simulink model "TEAM_6_MANUAL"  (R2020b)
settings: Solver=VariableStepAuto  StartTime=0.0  StopTime=10.0  RelTol=1e-3
libraries: simulink x2
settings Model: Creator=user  LastModifiedBy=99003740

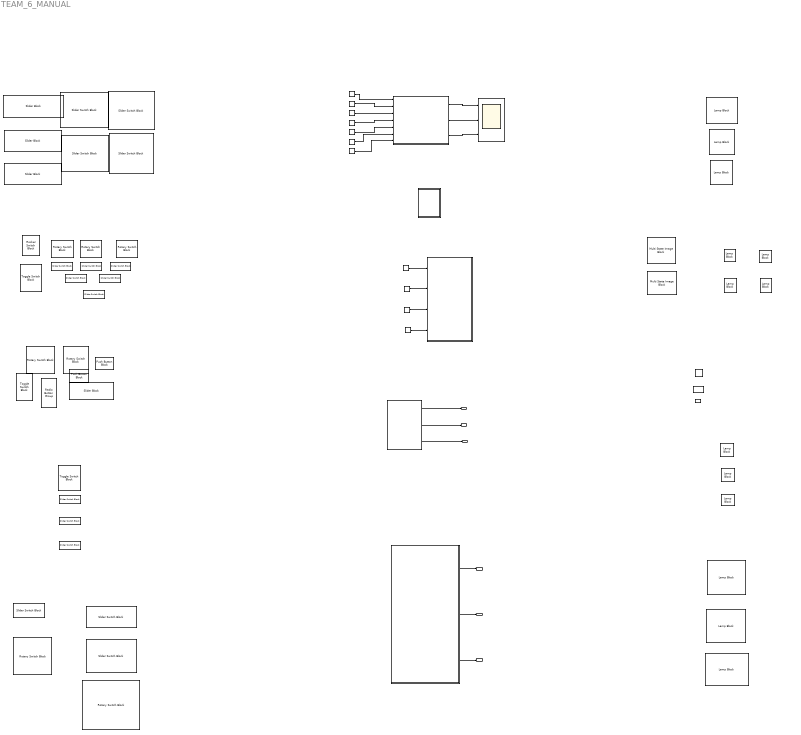
== system TEAM_6_MANUAL ==
  note: BCM_TEAM_6_HIL
  note: Wiper_band
  note: Dashboard
  note: KEY
  note: DASHBOARD
  note: DOME_LAMP
  note: Gray : Stop
      | Green : Very Slow
      | Blue : Normal Speed
      | Orange: Mid Speed
      | Yellow : High Speed
  note: BAT_Status
  note: Water_Spray
  note: Wiper
  note: Orange: Low BAT
      | Red : Very Low BAT
  note: READING_LAMP
  note: HVAC status Off
  note: WindShieldWiper
  note: Output Display
  note: Rear Fog removal OFF
  note: Air directed towards feet
  note: Air directed towards outlet
  note: Output Display
  note: HVAC status On
  note: Air directed towards windshield
  note: Recirculation
  note: Rear Fog removal ON
  " Passenger_Buckle" : SliderSwitchBlock
      settings: Values={{'Off', 'On'}, [0 1]}
  ACCESSORY : SliderSwitchBlock
      settings: Values={{'Off', 'On'}, [0 1]}
  BRIGHTNESS_BUTTON : RotarySwitchBlock
      settings: Values={{'Off', 'Low', 'Medium', 'High', 'very high'}, [0 1 2 3 4]}
  Bat : Constant  Value=24
  Controller : Subsystem
  DASHBOARD : LampBlock
  DOMELAMP : LampBlock
  DOME_BUTTON : SliderSwitchBlock
      settings: Values={{'Off', 'On'}, [0 1]}
  DOOR : RotarySwitchBlock
      settings: Values={{'Close', 'Door', 'Open'}, [0 1 2]}
  Driver remainder : LampBlock
  Driver_Buckle : SliderSwitchBlock
      settings: Values={{'Off', 'On'}, [0 1]}
  Front crash : Constant  Value=89.87630208333334
  Gear : Constant
  KEY : Constant  Value=0
  Lamp{,1..6} (7 alike) : LampBlock
  Lamp7 : LampBlock  LabelPosition=Hide
  Lamp8 : LampBlock  LabelPosition=Hide
  Lamp9 : LampBlock  LabelPosition=Hide
  MultiStateImage : MultiStateImageBlock
  MultiStateImage1 : MultiStateImageBlock
  Passenger Remainder : LampBlock
  Push Button : PushButtonBlock  LabelPosition=Bottom  ButtonText=Spray
  Push Button1 : PushButtonBlock  ButtonText=1X_Wiper
  READING_LAMP : LampBlock
  READLIGHT_BUTTON : SliderSwitchBlock
      settings: Values={{'Off', 'On'}, [0 1]}
  Radio Button : RadioButtonGroup  LabelPosition=Hide  SelectedLabel=P  ButtonGroupName=Gear_Box
      settings: Values={{'P', 'R', 'N', 'D', 'L'}, [1 2 0 3 4]}
  Rocker Switch : RockerSwitchBlock
      settings: Values={{'On', 'Off'}, [1 0]}
  Roll   Over : Constant  Value=73.98290094339622
  Rotary Switch : RotarySwitchBlock
      settings: Values={{'Off', 'Low', 'Medium', 'High'}, [0 1 2 3]}
  Rotary Switch1 : RotarySwitchBlock
      settings: Values={{'Off', 'Low', 'Medium', 'High'}, [0 1 2 3]}
  Rotary Switch2 : RotarySwitchBlock
      settings: Values={{'Off', 'AC', 'Heater', 'Air-Vent'}, [0 1 2 3]}
  Rotary Switch3 : RotarySwitchBlock  LabelPosition=Hide
      settings: Values={{'OFF', '-', 'NR', 'LO', 'HI'}, [0 1 2 3 4]}
  Rotary Switch4 : RotarySwitchBlock  LabelPosition=Hide
      settings: Values={{'OFF', 'ACC', 'IGNI'}, [0 1 2]}
  Scope1 : Scope  NumInputPorts=3
  Seatbelt{1..4} (4 alike) : Constant
  Side crash : Constant  Value=67.95726102941177
  Slider : SliderBlock
  Slider Switch{,1..6,9..12} (11 alike) : SliderSwitchBlock
      settings: Values={{'Off', 'On'}, [0 1]}
  Slider1 : SliderBlock
  Slider2 : SliderBlock
  Slider3 : SliderBlock  LabelPosition=Hide  ScaleMin=12  ScaleMax=24  TickInterval=6
  Subsystem1 : Subsystem
  Subsystem3 : Subsystem
  Subsystem4 : Subsystem
  Subsystem5 : Subsystem
  T_switch : Constant  Value=0
  Toggle Switch : ToggleSwitchBlock
      settings: Values={{'Off', 'On'}, [0 1]}
  Toggle Switch1 : ToggleSwitchBlock  LabelPosition=Hide
      settings: Values={{'TG_Close', 'TG_Open'}, [0 1]}
  Toggle Switch2 : ToggleSwitchBlock
      settings: Values={{'Off', 'On'}, [0 1]}
  Vehicle State : LampBlock
  Outport : Outport
  Outport1 : Outport  Port=2
  Outport2 : Outport  Port=3
  DL : Outport  Port=4
  dash_light : Outport  Port=5
  reading_lamp : Outport  Port=6
  wires:
  Side crash/1 -> Subsystem1/2(In2)
  Front crash/1 -> Subsystem1/1(In1)
  Seatbelt2/1 -> Subsystem1/5(Inport4)
  Subsystem1/3(All Airbag) -> Scope1/3
  Roll   Over/1 -> Subsystem1/3(Inport2)
  Seatbelt3/1 -> Subsystem1/6(Inport5)
  Seatbelt4/1 -> Subsystem1/7(Inport6)
  Subsystem1/2(Airbag Side) -> Scope1/2
  Seatbelt1/1 -> Subsystem1/4(Inport3)
  Subsystem1/1(Airbag front) -> Scope1/1
  Gear/1 -> Controller/2(GEAR)
  Bat/1 -> Controller/3(BAT)
  T_switch/1 -> Controller/4(T_Switch)
  KEY/1 -> Controller/1(KEY)
  Subsystem4/1(Outport) -> Outport/1
  Subsystem4/2(Outport1) -> Outport1/1
  Subsystem4/3(Outport2) -> Outport2/1
  Subsystem5/1(DL) -> DL/1
  Subsystem5/3(reading_lamp) -> reading_lamp/1
  Subsystem5/2(dash_light) -> dash_light/1

== system TEAM_6_MANUAL/Controller ==
  note: Wiper_system
  note: TailGate_System
  KEY : Inport
  GEAR : Inport  Port=2
  BAT : Inport  Port=3
  T_Switch : Inport  Port=4
  Tail_Gate : Subsystem
  Wiper_System : Subsystem
  wires:
  KEY/1 -> Wiper_System/2(KEY), Tail_Gate/1(KEY)
  GEAR/1 -> Tail_Gate/3(GEAR)  "gear"
  BAT/1 -> Tail_Gate/2(BAT), Wiper_System/1(BAT)  "bat"
  T_Switch/1 -> Tail_Gate/4(T_Switch)  "t_swiitch"

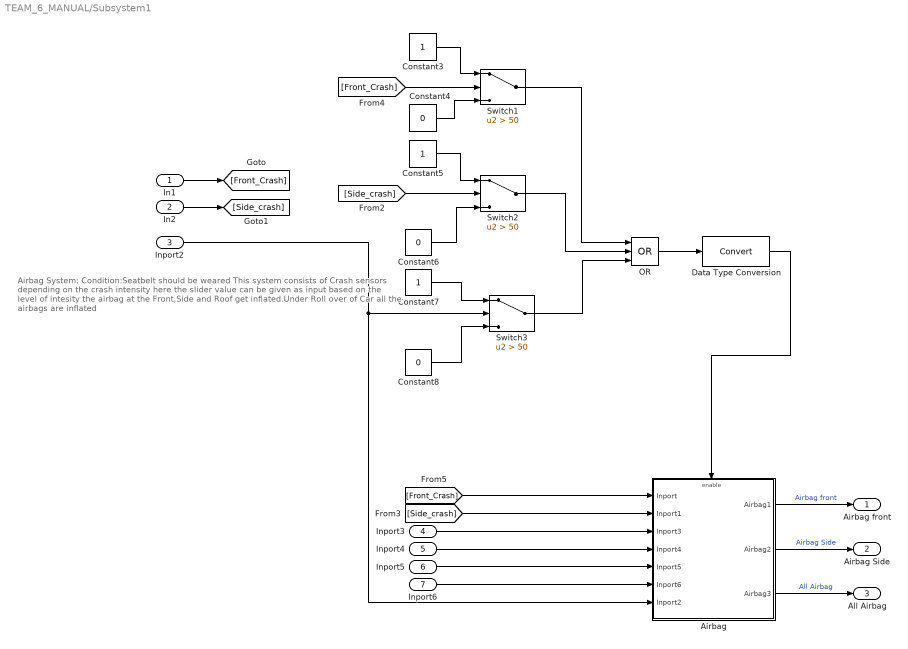
== system TEAM_6_MANUAL/Subsystem1 ==
  note: Airbag System:
      | Condition:Seatbelt should be weared
      | This system consists of Crash sensors depending on the
      | crash intensity here the slider value can be given as input
      | based on the level of intesity the airbag at the Front,Side and Roof get
      | inflated.Under Roll over of Car all the airbags are inflated
  In1 : Inport
  In2 : Inport  Port=2
  Inport2 : Inport  Port=3
  Inport3 : Inport  Port=4
  Inport4 : Inport  Port=5
  Inport5 : Inport  Port=6
  Inport6 : Inport  Port=7
  Airbag : Subsystem  TreatAsAtomicUnit=on
  Constant3 : Constant
  Constant4 : Constant  Value=0
  Constant5 : Constant
  Constant6 : Constant  Value=0
  Constant7 : Constant
  Constant8 : Constant  Value=0
  Data Type Conversion : DataTypeConversion
  OR : Logic  Operator=OR  Inputs=3  IconShape=distinctive  AllPortsSameDT=off  OutDataTypeStr=boolean
  Switch1 : Switch  Criteria=u2 > Threshold  Threshold=50
  Switch2 : Switch  Criteria=u2 > Threshold  Threshold=50
  Switch3 : Switch  Criteria=u2 > Threshold  Threshold=50
  Airbag front : Outport
  Airbag Side : Outport  Port=2
  All Airbag : Outport  Port=3
  wires:
  Constant7/1 -> Switch3/1
  Constant6/1 -> Switch2/3
  Switch3/1 -> OR/3
  Switch2/1 -> OR/2
  Airbag/3(Airbag3) -> All Airbag/1  "All Airbag"
  Airbag/2(Airbag2) -> Airbag Side/1  "Airbag Side"
  Inport6/1 -> Airbag/6(Inport6)
  OR/1 -> Data Type Conversion/1
  Inport4/1 -> Airbag/4(Inport4)
  Inport5/1 -> Airbag/5(Inport5)
  Inport2/1 -> Airbag/7(Inport2), Switch3/2
  In2/1 -> [Side_crash]
  [Side_crash] -> Airbag/2(Inport1)
  Constant4/1 -> Switch1/3
  [Front_Crash] -> Switch1/2
  [Front_Crash] -> Airbag/1(Inport)
  [Side_crash] -> Switch2/2
  Data Type Conversion/1 -> Airbag/Enable
  Constant3/1 -> Switch1/1
  In1/1 -> [Front_Crash]
  Switch1/1 -> OR/1
  Constant8/1 -> Switch3/3
  Constant5/1 -> Switch2/1
  Inport3/1 -> Airbag/3(Inport3)
  Airbag/1(Airbag1) -> Airbag front/1  "Airbag front"

== system TEAM_6_MANUAL/Subsystem3 ==
  note: HVAC SYSTEM
      |
      | Des cription:
  Hood and HVAC Subsystem : Subsystem  TreatAsAtomicUnit=on

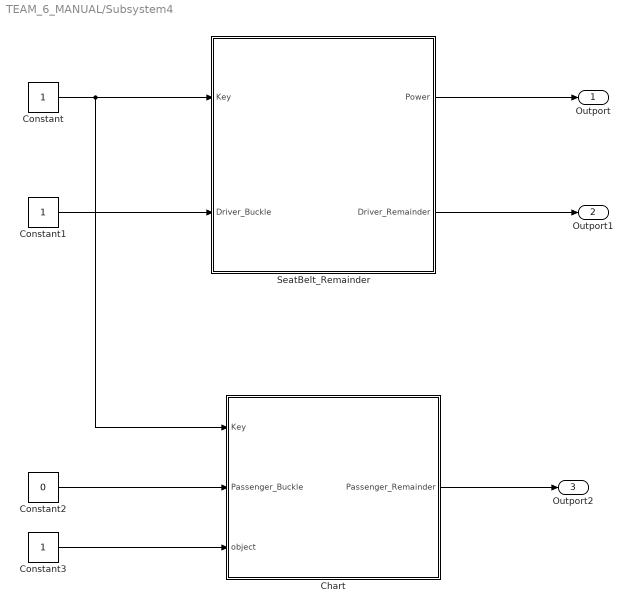
== system TEAM_6_MANUAL/Subsystem4 ==
  Chart : Stateflow chart  TreatAsAtomicUnit=on
  Constant : Constant
  Constant1 : Constant
  Constant2 : Constant  Value=0
  Constant3 : Constant
  SeatBelt_Remainder : Stateflow chart  TreatAsAtomicUnit=on
  Outport : Outport
  Outport1 : Outport  Port=2
  Outport2 : Outport  Port=3
  wires:
  Constant/1 -> Chart/1(Key), SeatBelt_Remainder/1(Key)
  SeatBelt_Remainder/1(Power) -> Outport/1
  SeatBelt_Remainder/2(Driver_Remainder) -> Outport1/1
  Constant1/1 -> SeatBelt_Remainder/2(Driver_Buckle)
  Constant2/1 -> Chart/2(Passenger_Buckle)
  Constant3/1 -> Chart/3(object)
  Chart/1(Passenger_Remainder) -> Outport2/1

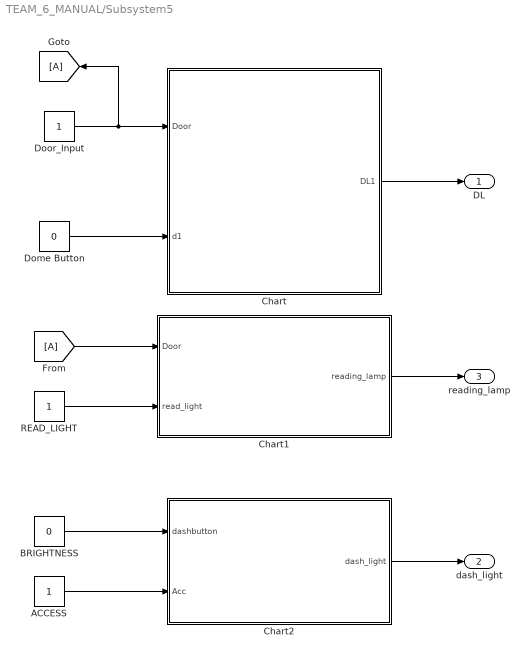
== system TEAM_6_MANUAL/Subsystem5 ==
  ACCESS : Constant
  BRIGHTNESS : Constant  Value=0
  Chart : Stateflow chart  TreatAsAtomicUnit=on
  Chart1 : Stateflow chart  TreatAsAtomicUnit=on
  Chart2 : Stateflow chart  TreatAsAtomicUnit=on
  Dome Button : Constant  Value=0
  Door_Input : Constant
  READ_LIGHT : Constant
  DL : Outport
  dash_light : Outport  Port=2
  reading_lamp : Outport  Port=3
  wires:
  Chart1/1(reading_lamp) -> reading_lamp/1
  Door_Input/1 -> Chart/1(Door), [A]
  [A] -> Chart1/1(Door)
  BRIGHTNESS/1 -> Chart2/1(dashbutton)
  ACCESS/1 -> Chart2/2(Acc)
  Chart2/1(dash_light) -> dash_light/1
  Chart/1(DL1) -> DL/1
  Dome Button/1 -> Chart/2(d1)
  READ_LIGHT/1 -> Chart1/2(read_light)

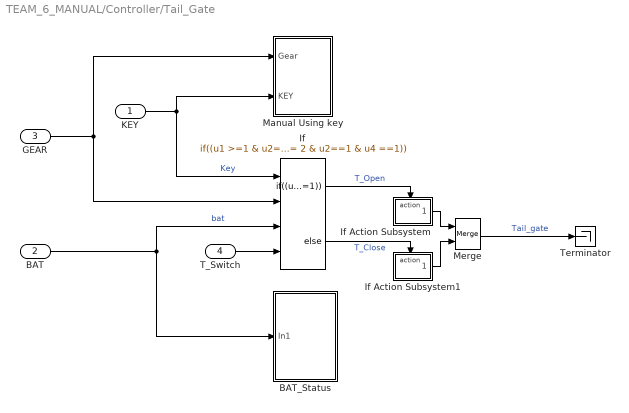
== system TEAM_6_MANUAL/Controller/Tail_Gate ==
  KEY : Inport
  BAT : Inport  Port=2
  GEAR : Inport  Port=3
  T_Switch : Inport  Port=4
  BAT_Status : Subsystem
  If : If  NumInputs=4  IfExpression=(u1 >=1 & u2==1 & u3 >20 & u4 ==1)|(u1 == 2 & u2==1 & u4 ==1)
  If Action Subsystem : Subsystem  TreatAsAtomicUnit=on
  If Action Subsystem1 : Subsystem  TreatAsAtomicUnit=on
  Manual Using key : Subsystem
  Merge : Merge
  Terminator : Terminator
  wires:
  If/1 -> If Action Subsystem/Action  "T_Open"
  BAT/1 -> If/3, BAT_Status/1(In1)  "bat"
  KEY/1 -> Manual Using key/2(KEY), If/1  "Key"
  GEAR/1 -> Manual Using key/1(Gear), If/2
  If Action Subsystem/1(Inport) -> Merge/1
  If/2 -> If Action Subsystem1/Action  "T_Close"
  If Action Subsystem1/1(Inport) -> Merge/2
  Merge/1 -> Terminator/1  "Tail_gate"
  T_Switch/1 -> If/4

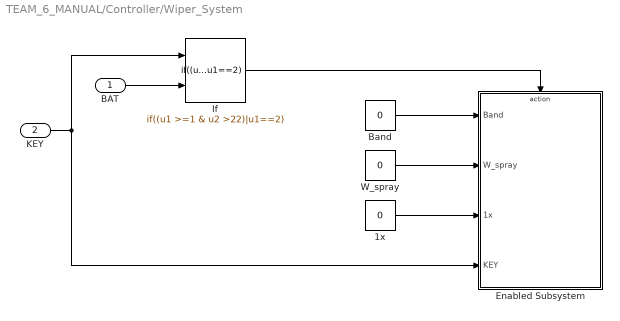
== system TEAM_6_MANUAL/Controller/Wiper_System ==
  BAT : Inport
  KEY : Inport  Port=2
  1x : Constant  Value=0
  Band : Constant  Value=0
  Enabled Subsystem : Subsystem  TreatAsAtomicUnit=on
  If : If  NumInputs=2  IfExpression=(u1 >=1 & u2 >22)|u1==2  ShowElse=off
  W_spray : Constant  Value=0
  wires:
  If/1 -> Enabled Subsystem/Action
  W_spray/1 -> Enabled Subsystem/2(W_spray)
  Band/1 -> Enabled Subsystem/1(Band)
  KEY/1 -> If/1, Enabled Subsystem/4(KEY)
  1x/1 -> Enabled Subsystem/3(1x)
  BAT/1 -> If/2

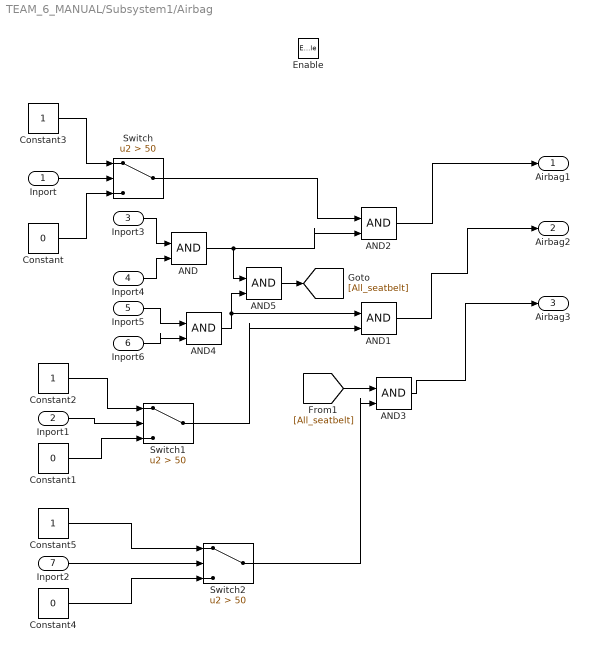
== system TEAM_6_MANUAL/Subsystem1/Airbag ==
  Inport : Inport
  Inport1 : Inport  Port=2
  Inport3 : Inport  Port=3
  Inport4 : Inport  Port=4
  Inport5 : Inport  Port=5
  Inport6 : Inport  Port=6
  Inport2 : Inport  Port=7
  Enable : EnablePort
  AND{,1..5} (6 alike) : Logic  IconShape=distinctive  AllPortsSameDT=off  OutDataTypeStr=boolean
  Constant : Constant  Value=0
  Constant1 : Constant  Value=0
  Constant2 : Constant
  Constant3 : Constant
  Constant4 : Constant  Value=0
  Constant5 : Constant
  Switch : Switch  Criteria=u2 > Threshold  Threshold=50
  Switch1 : Switch  Criteria=u2 > Threshold  Threshold=50
  Switch2 : Switch  Criteria=u2 > Threshold  Threshold=50
  Airbag1 : Outport
  Airbag2 : Outport  Port=2
  Airbag3 : Outport  Port=3
  wires:
  Constant2/1 -> Switch1/1
  Inport/1 -> Switch/2
  Constant/1 -> Switch/3
  Inport1/1 -> Switch1/2
  Constant1/1 -> Switch1/3
  Constant3/1 -> Switch/1
  Switch/1 -> AND2/1
  AND2/1 -> Airbag1/1
  AND1/1 -> Airbag2/1
  AND3/1 -> Airbag3/1
  Inport3/1 -> AND/1
  Inport4/1 -> AND/2
  Inport5/1 -> AND4/1
  Inport6/1 -> AND4/2
  Constant4/1 -> Switch2/3
  Inport2/1 -> Switch2/2
  Constant5/1 -> Switch2/1
  AND/1 -> AND5/1, AND2/2
  AND4/1 -> AND1/1, AND5/2
  Switch1/1 -> AND1/2
  AND5/1 -> [All_seatbelt]
  [All_seatbelt] -> AND3/1
  Switch2/1 -> AND3/2

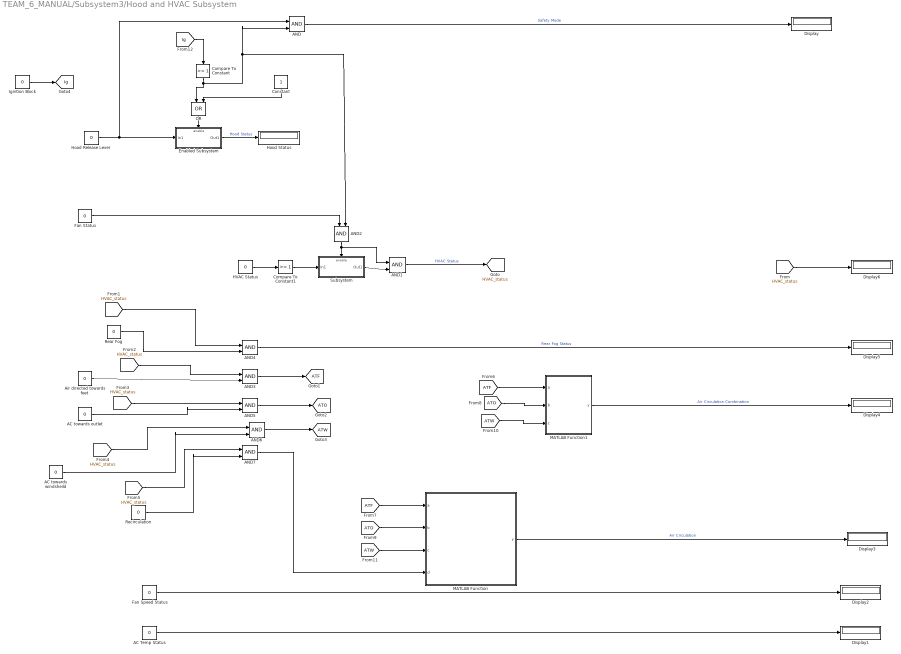
== system TEAM_6_MANUAL/Subsystem3/Hood and HVAC Subsystem ==
  AC Temp Status : Constant  Value=0
  AC towards outlet : Constant  Value=0
  AC towards windsheild : Constant  Value=0
  AND{,1..7} (8 alike) : Logic  IconShape=distinctive  AllPortsSameDT=off  OutDataTypeStr=boolean
  Air directed towards feet : Constant  Value=0
  Compare To Constant : simulink/Logic and Bit Operations/Compare To Constant  relop=>=  const=1  OutDataTypeStr=boolean
  Compare To Constant1 : simulink/Logic and Bit Operations/Compare To Constant  relop=>=  const=1  OutDataTypeStr=boolean
  Constant : Constant
  Display{,1..6} (7 alike) : Display
  Enabled Subsystem : Subsystem  TreatAsAtomicUnit=on
  Fan Speed Status : Constant  Value=0
  Fan Status : Constant  Value=0
  HVAC Status : Constant  Value=0
  Hood Release Lever : Constant  Value=0
  Hood Status : Display
  Ignition Block : Constant  Value=0
  MATLAB Function : MATLAB Function  TreatAsAtomicUnit=on
  MATLAB Function1 : MATLAB Function  TreatAsAtomicUnit=on
  OR : Logic  Operator=OR  IconShape=distinctive  AllPortsSameDT=off  OutDataTypeStr=boolean
  Rear Fog : Constant  Value=0
  Recirculation : Constant  Value=0
  Subsystem : Subsystem
  tag scope: ATF=global, ATO=global, ATW=global, HVAC_status=global, Ig=global
  wires:
  AND/1 -> Display/1  "Safety Mode"
  Hood Release Lever/1 -> Enabled Subsystem/1(In1), AND/1
  Compare To Constant/1 -> AND2/2, AND/2, OR/1
  OR/1 -> Enabled Subsystem/Enable
  Enabled Subsystem/1(Out1) -> Hood Status/1  "Hood Status"
  Constant/1 -> OR/2
  AND1/1 -> [HVAC_status]  "HVAC Status"
  Subsystem/1(Out1) -> AND1/2
  AND2/1 -> AND1/1, Subsystem/Enable
  Compare To Constant1/1 -> Subsystem/1(In1)
  HVAC Status/1 -> Compare To Constant1/1
  Recirculation/1 -> AND7/2
  AND4/1 -> Display5/1  "Rear Fog Status"
  Rear Fog/1 -> AND4/2
  AC towards outlet/1 -> AND5/2
  Air directed towards feet/1 -> AND3/2
  AC towards windsheild/1 -> AND6/2
  MATLAB Function/1(y) -> Display3/1  "Air Circulation"
  AND7/1 -> MATLAB Function/4(d)
  MATLAB Function1/1(y) -> Display4/1  "Air Circulation Combination"
  AC Temp Status/1 -> Display1/1
  Fan Speed Status/1 -> Display2/1
  Fan Status/1 -> AND2/1
  [HVAC_status] -> Display6/1
  [HVAC_status] -> AND4/1
  [HVAC_status] -> AND3/1
  [HVAC_status] -> AND5/1
  [HVAC_status] -> AND6/1
  [HVAC_status] -> AND7/1
  AND3/1 -> [ATF]
  [ATF] -> MATLAB Function1/1(a)
  [ATF] -> MATLAB Function/1(a)
  AND5/1 -> [ATO]
  [ATO] -> MATLAB Function1/2(b)
  [ATO] -> MATLAB Function/2(b)
  AND6/1 -> [ATW]
  [ATW] -> MATLAB Function1/3(c)
  [ATW] -> MATLAB Function/3(c)
  Ignition Block/1 -> [Ig]
  [Ig] -> Compare To Constant/1

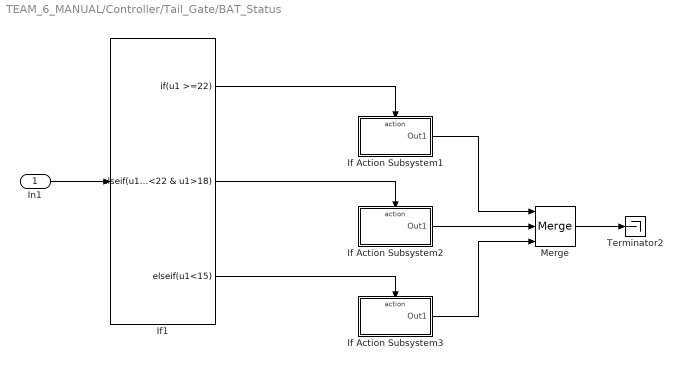
== system TEAM_6_MANUAL/Controller/Tail_Gate/BAT_Status ==
  In1 : Inport
  If Action Subsystem1 : Subsystem  TreatAsAtomicUnit=on
  If Action Subsystem2 : Subsystem  TreatAsAtomicUnit=on
  If Action Subsystem3 : Subsystem  TreatAsAtomicUnit=on
  If1 : If  IfExpression=u1 >=22  ElseIfExpressions=u1<22 & u1>18, u1<15  ShowElse=off
  Merge : Merge  Inputs=3
  Terminator2 : Terminator
  wires:
  In1/1 -> If1/1
  If Action Subsystem1/1(Out1) -> Merge/1
  Merge/1 -> Terminator2/1
  If1/1 -> If Action Subsystem1/Action
  If1/2 -> If Action Subsystem2/Action
  If Action Subsystem3/1(Out1) -> Merge/3
  If1/3 -> If Action Subsystem3/Action
  If Action Subsystem2/1(Out1) -> Merge/2

== system TEAM_6_MANUAL/Controller/Tail_Gate/If Action Subsystem ==
  Action Port : ActionPort  ActionPortLabel=if((u1 >=1 & u2==1 & u3 >20 & u4 ==1)|(u1 == 2 & u2==1 & u4 ==1))
  Constant : Constant
  Inport : Outport
  wires:
  Constant/1 -> Inport/1

== system TEAM_6_MANUAL/Controller/Tail_Gate/If Action Subsystem1 ==
  Action Port : ActionPort  ActionPortLabel=else
  Constant : Constant  Value=0
  Inport : Outport
  wires:
  Constant/1 -> Inport/1

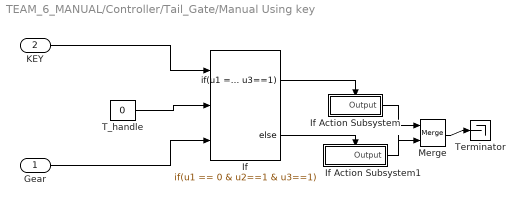
== system TEAM_6_MANUAL/Controller/Tail_Gate/Manual Using key ==
  Gear : Inport
  KEY : Inport  Port=2
  If : If  NumInputs=3  IfExpression=u1 == 0 & u2==1 & u3==1
  If Action Subsystem : Subsystem  TreatAsAtomicUnit=on
  If Action Subsystem1 : Subsystem  TreatAsAtomicUnit=on
  Merge : Merge
  T_handle : Constant  Value=0
  Terminator : Terminator
  wires:
  KEY/1 -> If/1
  If Action Subsystem/1(Output) -> Merge/1
  If/1 -> If Action Subsystem/Action
  If Action Subsystem1/1(Output) -> Merge/2
  If/2 -> If Action Subsystem1/Action
  Merge/1 -> Terminator/1
  T_handle/1 -> If/2
  Gear/1 -> If/3

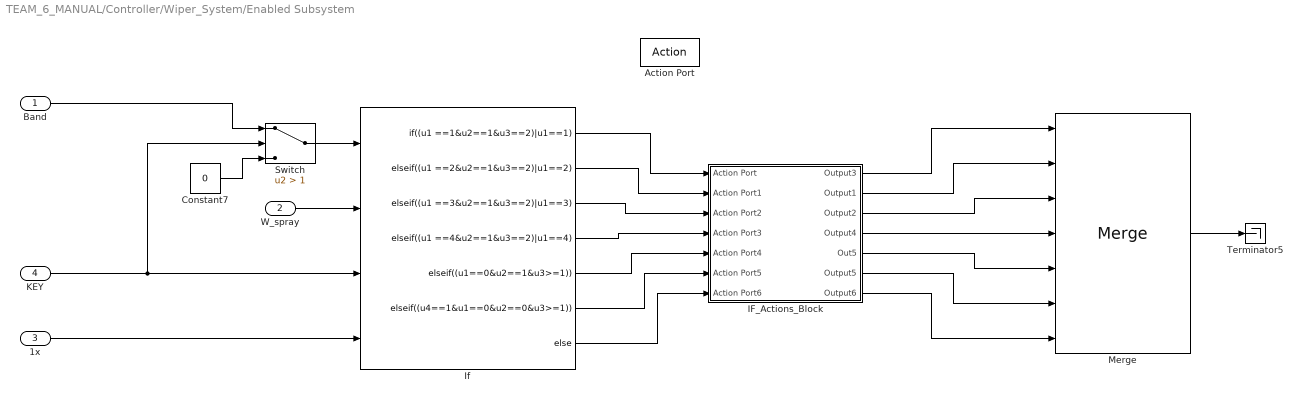
== system TEAM_6_MANUAL/Controller/Wiper_System/Enabled Subsystem ==
  Band : Inport
  W_spray : Inport  Port=2
  1x : Inport  Port=3
  KEY : Inport  Port=4
  Action Port : ActionPort  ActionPortLabel=if((u1 >=1 & u2 >22)|u1==2)
  Constant7 : Constant  Value=0
  IF_Actions_Block : Subsystem
  If : If  NumInputs=4  IfExpression=(u1 ==1&u2==1&u3==2)|u1==1  ElseIfExpressions=(u1 ==2&u2==1&u3==2)|u1==2,(u1 ==3&u2==1&u3==2)|u1==3,(u1 ==4&u2==1&u3==2)|u1==4,(u1==0&u2==1&u3>=1),(u4==1&u1==0&u2==0&u3>=1)
  Merge : Merge  Inputs=7
  Switch : Switch  Criteria=u2 > Threshold  Threshold=1
  Terminator5 : Terminator
  wires:
  Merge/1 -> Terminator5/1
  W_spray/1 -> If/2
  1x/1 -> If/4
  KEY/1 -> Switch/2, If/3
  Switch/1 -> If/1
  Band/1 -> Switch/1
  Constant7/1 -> Switch/3
  If/1 -> IF_Actions_Block/1(Action Port)
  If/2 -> IF_Actions_Block/2(Action Port1)
  If/3 -> IF_Actions_Block/3(Action Port2)
  If/4 -> IF_Actions_Block/4(Action Port3)
  If/5 -> IF_Actions_Block/5(Action Port4)
  If/6 -> IF_Actions_Block/6(Action Port5)
  If/7 -> IF_Actions_Block/7(Action Port6)
  IF_Actions_Block/1(Output3) -> Merge/1
  IF_Actions_Block/2(Output1) -> Merge/2
  IF_Actions_Block/3(Output2) -> Merge/3
  IF_Actions_Block/4(Output4) -> Merge/4
  IF_Actions_Block/5(Out5) -> Merge/5
  IF_Actions_Block/6(Output5) -> Merge/6
  IF_Actions_Block/7(Output6) -> Merge/7

== system TEAM_6_MANUAL/Subsystem3/Hood and HVAC Subsystem/Enabled Subsystem ==
  In1 : Inport
  Enable : EnablePort
  Out1 : Outport  InitialOutput=0  VectorParamsAs1DForOutWhenUnconnected=off
  wires:
  In1/1 -> Out1/1

== system TEAM_6_MANUAL/Subsystem3/Hood and HVAC Subsystem/Subsystem ==
  In1 : Inport
  Enable : EnablePort
  Out1 : Outport
  wires:
  In1/1 -> Out1/1

== system TEAM_6_MANUAL/Controller/Tail_Gate/BAT_Status/If Action Subsystem1 ==
  Action Port : ActionPort  ActionPortLabel=if(u1 >=22)
  Constant : Constant
  Out1 : Outport
  wires:
  Constant/1 -> Out1/1

== system TEAM_6_MANUAL/Controller/Tail_Gate/BAT_Status/If Action Subsystem2 ==
  Action Port : ActionPort  ActionPortLabel=elseif(u1<22 & u1>18)
  Constant : Constant  Value=2
  Out1 : Outport
  wires:
  Constant/1 -> Out1/1

== system TEAM_6_MANUAL/Controller/Tail_Gate/BAT_Status/If Action Subsystem3 ==
  Action Port : ActionPort  ActionPortLabel=elseif( u1<15)
  Constant : Constant  Value=3
  Out1 : Outport
  wires:
  Constant/1 -> Out1/1

== system TEAM_6_MANUAL/Controller/Tail_Gate/Manual Using key/If Action Subsystem ==
  Action Port : ActionPort  ActionPortLabel=if(u1 == 0 & u2==1 & u3==1)
  Constant2 : Constant
  Output : Outport
  wires:
  Constant2/1 -> Output/1

== system TEAM_6_MANUAL/Controller/Tail_Gate/Manual Using key/If Action Subsystem1 ==
  Action Port : ActionPort  ActionPortLabel=else
  Constant3 : Constant  Value=0
  Output : Outport
  wires:
  Constant3/1 -> Output/1

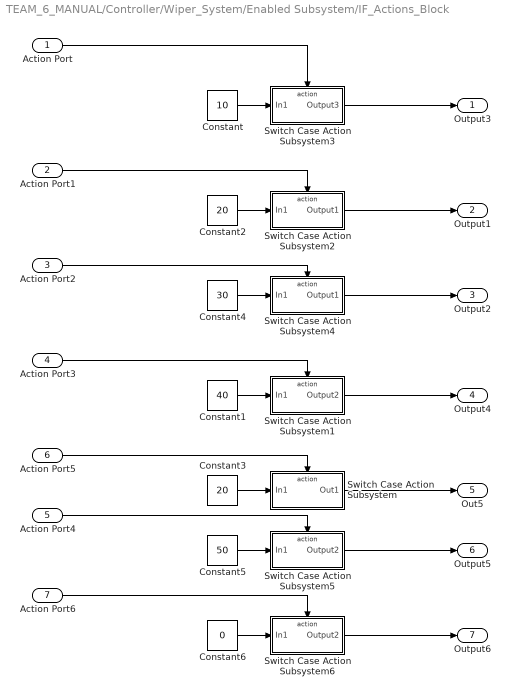
== system TEAM_6_MANUAL/Controller/Wiper_System/Enabled Subsystem/IF_Actions_Block ==
  Action Port : Inport
  Action Port1 : Inport  Port=2
  Action Port2 : Inport  Port=3
  Action Port3 : Inport  Port=4
  Action Port4 : Inport  Port=5
  Action Port5 : Inport  Port=6
  Action Port6 : Inport  Port=7
  Constant : Constant  Value=10
  Constant1 : Constant  Value=40
  Constant2 : Constant  Value=20
  Constant3 : Constant  Value=20
  Constant4 : Constant  Value=30
  Constant5 : Constant  Value=50
  Constant6 : Constant  Value=0
  Switch Case Action Subsystem : Subsystem  TreatAsAtomicUnit=on
  Switch Case Action Subsystem1 : Subsystem  TreatAsAtomicUnit=on
  Switch Case Action Subsystem2 : Subsystem  TreatAsAtomicUnit=on
  Switch Case Action Subsystem3 : Subsystem  TreatAsAtomicUnit=on
  Switch Case Action Subsystem4 : Subsystem  TreatAsAtomicUnit=on
  Switch Case Action Subsystem5 : Subsystem  TreatAsAtomicUnit=on
  Switch Case Action Subsystem6 : Subsystem  TreatAsAtomicUnit=on
  Output3 : Outport
  Output1 : Outport  Port=2
  Output2 : Outport  Port=3
  Output4 : Outport  Port=4
  Out5 : Outport  Port=5
  Output5 : Outport  Port=6
  Output6 : Outport  Port=7
  wires:
  Action Port2/1 -> Switch Case Action Subsystem4/Action
  Switch Case Action Subsystem4/1(Output1) -> Output2/1
  Constant4/1 -> Switch Case Action Subsystem4/1(In1)
  Switch Case Action Subsystem3/1(Output3) -> Output3/1
  Constant6/1 -> Switch Case Action Subsystem6/1(In1)
  Switch Case Action Subsystem2/1(Output1) -> Output1/1
  Switch Case Action Subsystem1/1(Output2) -> Output4/1
  Constant3/1 -> Switch Case Action Subsystem/1(In1)
  Action Port1/1 -> Switch Case Action Subsystem2/Action
  Constant/1 -> Switch Case Action Subsystem3/1(In1)
  Constant1/1 -> Switch Case Action Subsystem1/1(In1)
  Action Port/1 -> Switch Case Action Subsystem3/Action
  Switch Case Action Subsystem/1(Out1) -> Out5/1
  Constant5/1 -> Switch Case Action Subsystem5/1(In1)
  Switch Case Action Subsystem5/1(Output2) -> Output5/1
  Constant2/1 -> Switch Case Action Subsystem2/1(In1)
  Action Port4/1 -> Switch Case Action Subsystem5/Action
  Action Port3/1 -> Switch Case Action Subsystem1/Action
  Action Port5/1 -> Switch Case Action Subsystem/Action
  Action Port6/1 -> Switch Case Action Subsystem6/Action
  Switch Case Action Subsystem6/1(Output2) -> Output6/1

== system TEAM_6_MANUAL/Controller/Wiper_System/Enabled Subsystem/IF_Actions_Block/Switch Case Action Subsystem ==
  In1 : Inport
  Action Port : ActionPort  ActionPortLabel=elseif((u4==1&u1==0&u2==0&u3>=1))
  Out1 : Outport
  wires:
  In1/1 -> Out1/1

== system TEAM_6_MANUAL/Controller/Wiper_System/Enabled Subsystem/IF_Actions_Block/Switch Case Action Subsystem1 ==
  In1 : Inport
  Action Port : ActionPort  ActionPortLabel=elseif((u1 ==4&u2==1&u3==2)|u1==4)
  Output2 : Outport
  wires:
  In1/1 -> Output2/1

== system TEAM_6_MANUAL/Controller/Wiper_System/Enabled Subsystem/IF_Actions_Block/Switch Case Action Subsystem2 ==
  In1 : Inport
  Action Port : ActionPort  ActionPortLabel=elseif((u1 ==2&u2==1&u3==2)|u1==2)
  Output1 : Outport
  wires:
  In1/1 -> Output1/1

== system TEAM_6_MANUAL/Controller/Wiper_System/Enabled Subsystem/IF_Actions_Block/Switch Case Action Subsystem3 ==
  In1 : Inport
  Action Port : ActionPort  ActionPortLabel=if((u1 ==1&u2==1&u3==2)|u1==1)
  Output3 : Outport
  wires:
  In1/1 -> Output3/1

== system TEAM_6_MANUAL/Controller/Wiper_System/Enabled Subsystem/IF_Actions_Block/Switch Case Action Subsystem4 ==
  In1 : Inport
  Action Port : ActionPort  ActionPortLabel=elseif((u1 ==3&u2==1&u3==2)|u1==3)
  Output1 : Outport
  wires:
  In1/1 -> Output1/1

== system TEAM_6_MANUAL/Controller/Wiper_System/Enabled Subsystem/IF_Actions_Block/Switch Case Action Subsystem5 ==
  In1 : Inport
  Action Port : ActionPort  ActionPortLabel=elseif((u1==0&u2==1&u3>=1))
  Output2 : Outport
  wires:
  In1/1 -> Output2/1

== system TEAM_6_MANUAL/Controller/Wiper_System/Enabled Subsystem/IF_Actions_Block/Switch Case Action Subsystem6 ==
  In1 : Inport
  Action Port : ActionPort  ActionPortLabel=else
  Output2 : Outport
  wires:
  In1/1 -> Output2/1

== matlab function TEAM_6_MANUAL/Subsystem3/Hood and HVAC Subsystem/MATLAB Function ==
  data: a input; b input; y output; c input; d input
function y = fcn(a, b, c, d)
    if a==1 && b==0 && c==0 && d==0
        y=1;
    elseif a==0 && b==1 &&c==0 && d==0
        y=2;
    elseif a==0 && b==0 &&c==1 && d==0
        y=3;
    elseif a==0 && b==0 &&c==0 && d==1
        y=4;
    else
        y=0;
    end
    

end

== stateflow chart TEAM_6_MANUAL/Subsystem4/Chart ==
  state passenger_state
    entry:
    Power=0;
    Passenger_Remainder=0;
  state remainder
    entry:
    Passenger_Remainder = 0;
  state object_detection
    entry:
    Power=1;
    Passenger_Remainder=0;
  state Object
    entry:
    Passenger_Remainder =1;
  remainder -> passenger_state [order 1] : [Key == 0]
  Object -> passenger_state [order 3] : [Key == 0]
  (default) -> passenger_state
  Object -> remainder [order 1] : [Passenger_Buckle == 1]
  object_detection -> passenger_state [order 1] : [Key == 0 ]
  object_detection -> Object [order 2] : [object == 1]
  remainder -> Object [order 2] : [Passenger_Buckle == 0]
  passenger_state -> object_detection : [ Key== 1 ]
  Object -> object_detection [order 2] : [object == 0]
  data: Key input; Passenger_Buckle input; Passenger_Remainder output; object input; Power local

== stateflow chart TEAM_6_MANUAL/Subsystem4/SeatBelt_Remainder ==
  state Indicator
    entry:
    Power=1;
    Driver_Remainder=1 ;
  state VehicleOff
    entry:
    Power=0;
    Driver_Remainder=0;
  state SeatBeltBuckled
    entry:
    Driver_Remainder=0;
  SeatBeltBuckled -> VehicleOff [order 2] : [Key == 0]
  (default) -> VehicleOff
  Indicator -> SeatBeltBuckled [order 1] : [Driver_Buckle==1]
  Indicator -> VehicleOff [order 2] : after(5,sec) [Key==0]
  SeatBeltBuckled -> Indicator [order 1] : [Driver_Buckle == 0]
  VehicleOff -> Indicator : [Key==1 ]
  data: Power output; Key input =0; Driver_Buckle input; Driver_Remainder output

== stateflow chart TEAM_6_MANUAL/Subsystem5/Chart ==
  state Default
    entry:
    DL1=0;
  state LightOn
    entry:
    DL1=1;
  (default) -> Default
  LightOn -> Default : [Door==0||(Door==1&&(d1==0))]
  Default -> LightOn : [Door==2||(Door==1&&(d1==1))]
  data: Door input; d1 input; DL1 output

== stateflow chart TEAM_6_MANUAL/Subsystem5/Chart1 ==
  state readlampon
    entry:
    reading_lamp=0;
  state readlampoff
    entry:
    reading_lamp=1;
  (default) -> readlampon
  readlampoff -> readlampon : [Door==0||(Door==1&&read_light==0)]
  readlampon -> readlampoff : [Door==2||(Door==1&&read_light==1)]
  data: Door input; read_light input; reading_lamp output

== stateflow chart TEAM_6_MANUAL/Subsystem5/Chart2 ==
  state dashboard_brightness
    entry:
    dash_light=0;
  state dashboard_brightness1
    entry:
    dash_light=1;
  state dashboard_brightness2
    entry:
    dash_light=2;
  state dashboard_brightness3
    entry:
    dash_light=3;
  state dashboard_brightness4
    entry:
    dash_light=4;
  (default) -> dashboard_brightness
  dashboard_brightness1 -> dashboard_brightness2 [order 1] : [dashbutton==2&&Acc==1]
  dashboard_brightness2 -> dashboard_brightness3 [order 1] : [dashbutton==3&&Acc==1]
  dashboard_brightness -> dashboard_brightness1 : [dashbutton==1&&Acc==1]
  dashboard_brightness3 -> dashboard_brightness4 [order 1] : [dashbutton==4&&Acc==1]
  dashboard_brightness2 -> dashboard_brightness1 [order 2] : [dashbutton==1&&Acc==1]
  dashboard_brightness3 -> dashboard_brightness2 [order 2] : [dashbutton == 2&&Acc==1]
  dashboard_brightness4 -> dashboard_brightness3 : [dashbutton==3&&Acc==1]
  dashboard_brightness1 -> dashboard_brightness [order 2] : [dashbutton==0&&Acc==1]
  data: dash_light output; dashbutton input; Acc input

== matlab function TEAM_6_MANUAL/Subsystem3/Hood and HVAC Subsystem/MATLAB Function1 ==
  data: a input; b input; c input; y output
function y = fcn(a,b,c)
    if a==1&& b==1 && c==1
        y=1;
    elseif a==1 && b==1 && c==0
        y=2;
    elseif a==1 && b==0 && c==1
        y=3;
    elseif a==0 && b==1 && c==1
        y=4;
    else
        y=0;
    end

end
